simulink model "State_Feedback_Controller"  (R2020b)
settings: Solver=VariableStepAuto  StartTime=0.0  StopTime=3  RelTol=1e-3
settings Model: Creator=Kevin  LastModifiedBy=Kevin

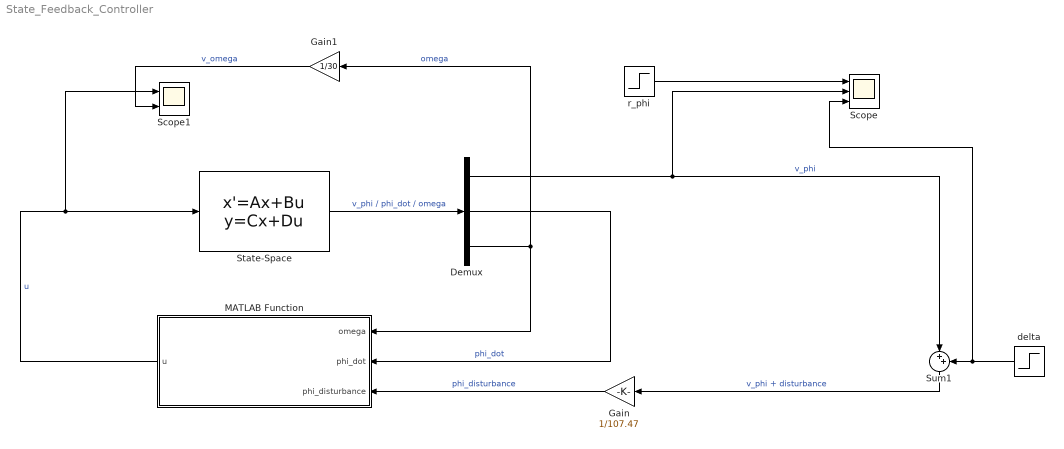
== system State_Feedback_Controller ==
  Demux : Demux  Outputs=3
  Gain : Gain  Gain=1/107.47
  Gain1 : Gain  Gain=1/30
  MATLAB Function : MATLAB Function  TreatAsAtomicUnit=on
  Scope : Scope  NumInputPorts=3
  Scope1 : Scope  NumInputPorts=2
  State-Space : StateSpace  A=[0 1 0; 23.5031 0 0.0045; -23.5031 0 -19.9513]  B=[0; 0.1393; -621.6819]  C=[107.47 0 0; 0 1 0; 0 0 1]  D=[0; 0; 0]  InitialCondition=[0.001860984460780 0 0]
  Sum1 : Sum  Inputs=|++
  delta : Step  Time=1.5  After=0.2  SampleTime=0
  r_phi : Step  Time=0  After=0  SampleTime=0
  wires:
  r_phi/1 -> Scope/1
  Gain/1 -> MATLAB Function/3(phi_disturbance)  "phi_disturbance"
  Demux/1 -> Scope/2, Sum1/1  "v_phi"
  Demux/2 -> MATLAB Function/2(phi_dot)  "phi_dot"
  State-Space/1 -> Demux/1  "v_phi / phi_dot / omega"
  Sum1/1 -> Gain/1  "v_phi + disturbance"
  Demux/3 -> Gain1/1, MATLAB Function/1(omega)  "omega"
  delta/1 -> Scope/3, Sum1/2
  MATLAB Function/1(u) -> Scope1/1, State-Space/1  "u"
  Gain1/1 -> Scope1/2  "v_omega"

== matlab function State_Feedback_Controller/MATLAB Function ==
  data: omega input; phi_dot input; phi_disturbance input; u output
function u = state_feedback_control_law(omega, phi_dot, phi_disturbance)

K = [2290 472 0.0771];
x = [phi_disturbance; phi_dot; omega];

u = -K*x;
